simulink model "HighwayLaneFollowingTestBench"  (R2020a)
settings: Solver=ode23tb  StartTime=0.0  StopTime=scenario.StopTime  RelTol=1e-3
PostLoadFcn:
  | helperSLHighwayLaneFollowingSetup
values from neighbouring files (symbols this model uses):
  camera = obj.Camera    [HelperLaneMarkerDetector.m]    (also in HelperVisionVehicleDetector.m)
  m = hActors.Actors(n).ActorID.Data(sampleIndex)    [helperPlotLFDetectionResults.m]
  scenario = drivingScenario    [helperGetLaneFollowingScenario.m]
  vehSim3D = repmat(     struct(         'Length', 0,         'RearOverhang', 0,         'InitialPos',[0 0 0],         'InitialRot',[0 0 0]),     numVehicles,1)    [helperSLHighwayLaneFollowingSetup.m]
undefined symbols (not defined in the file or in its folder): actorProfiles, assessment, driving, lr, max_ac, max_dc, tau, tau2, Ts, v_set
libraries: drivingscenarioandsensors x9, sim3dautolib x6, simulink x4, helperCoordinateTransformLib x1, sim3dcameralib x1, sim3dprobsensorlib x1, sim3dlib x1, dspvision x1, autolibshared x1
CloseFcn:
  | helperSLHighwayLaneFollowingCleanUp
settings Model: SILPILModeSetting=veronly  SILPILSystemUnderTest=refmodels  Creator=The MathWorks, Inc.  LastModifiedBy=The MathWorks, Inc.
settings DataIOCC: SaveOutput=off  SaveTime=off  ReturnWorkspaceOutputs=off
settings DebuggingCC: ParameterPrecisionLossMsg=none  PregeneratedLibrarySubsystemCodeDiagnostic=none  ArithmeticOperatorsInVariantConditions=warning
settings HardwareCC: ProdLongLongMode=on
settings SFSimCC: SimUseLocalCustomCode=off
settings RTWCC: RTWUseLocalCustomCode=off
settings GRTTargetCC: RTWCAPISignals=on
settings ConfigComp: CovScope=ReferencedModels  CovIncludeTopModel=off

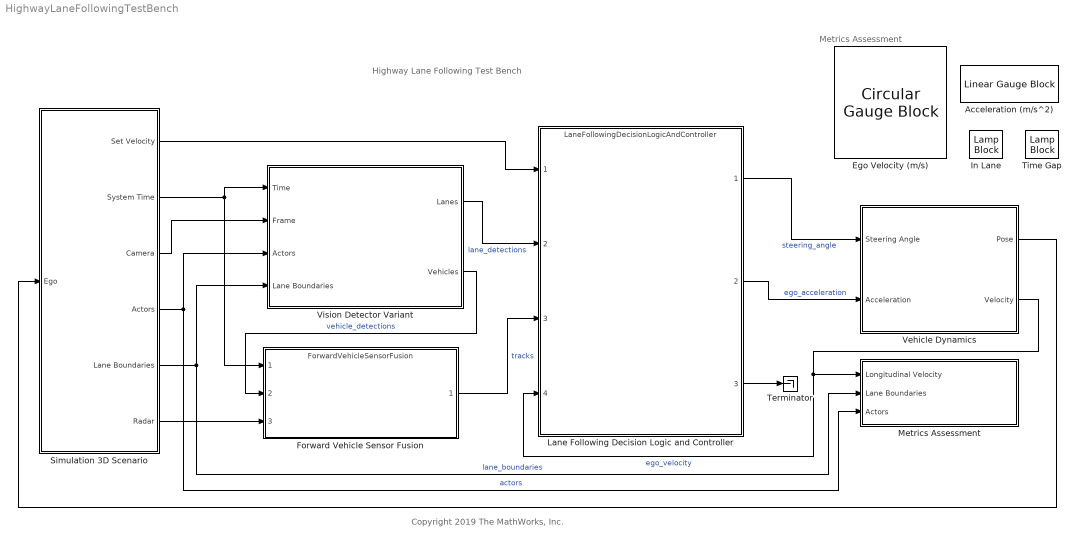
== system HighwayLaneFollowingTestBench ==
  note: Highway Lane Following Test Bench
  note: Metrics Assessment
  note: Copyright 2019 The MathWorks, Inc.
  Acceleration (m/s^2) : LinearGaugeBlock  LabelPosition=Hide  ScaleMin=-6  ScaleMax=6
  Ego Velocity (m/s) : CircularGaugeBlock  LabelPosition=Hide  ScaleMax=50
  Forward Vehicle Sensor Fusion : ModelReference  ModelNameDialog=ForwardVehicleSensorFusion.slx  SimulationMode=Normal  CodeInterface=Top model  ModelReferenceVersion=1.1423
  In Lane : LampBlock  LabelPosition=Hide
  Lane Following Decision Logic and Controller : ModelReference  ModelNameDialog=LaneFollowingDecisionLogicAndController.slx  SimulationMode=Normal  CodeInterface=Top model  ModelReferenceVersion=1.819
  Metrics Assessment : Subsystem
  Simulation 3D Scenario : Subsystem  VariantControl=1
  Terminator : Terminator
  Time Gap : LampBlock  LabelPosition=Hide
  Vehicle Dynamics : Subsystem  VariantControl=Variant2
  Vision Detector Variant : Subsystem  Variant=on
  wires:
  Vehicle Dynamics/2(Velocity) -> Metrics Assessment/1(Longitudinal Velocity), Lane Following Decision Logic and Controller/4  "ego_velocity"
  Simulation 3D Scenario/3(Camera) -> Vision Detector Variant/2(Frame)
  Simulation 3D Scenario/2(System Time) -> Vision Detector Variant/1(Time), Forward Vehicle Sensor Fusion/1
  Vehicle Dynamics/1(Pose) -> Simulation 3D Scenario/1(Ego)
  Simulation 3D Scenario/5(Lane Boundaries) -> Vision Detector Variant/4(Lane Boundaries), Metrics Assessment/2(Lane Boundaries)  "lane_boundaries"
  Simulation 3D Scenario/4(Actors) -> Metrics Assessment/3(Actors), Vision Detector Variant/3(Actors)  "actors"
  Lane Following Decision Logic and Controller/1 -> Vehicle Dynamics/1(Steering Angle)  "steering_angle"
  Simulation 3D Scenario/1(Set Velocity) -> Lane Following Decision Logic and Controller/1
  Lane Following Decision Logic and Controller/2 -> Vehicle Dynamics/2(Acceleration)  "ego_acceleration"
  Lane Following Decision Logic and Controller/3 -> Terminator/1
  Vision Detector Variant/1(Lanes) -> Lane Following Decision Logic and Controller/2  "lane_detections"
  Forward Vehicle Sensor Fusion/1 -> Lane Following Decision Logic and Controller/3  "tracks"
  Vision Detector Variant/2(Vehicles) -> Forward Vehicle Sensor Fusion/2  "vehicle_detections"
  Simulation 3D Scenario/6(Radar) -> Forward Vehicle Sensor Fusion/3

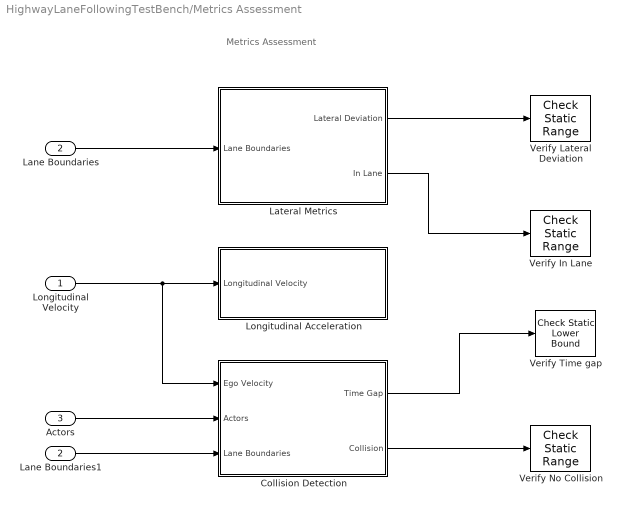
== system HighwayLaneFollowingTestBench/Metrics Assessment ==
  note: Metrics Assessment
  Longitudinal Velocity : Inport
  Lane Boundaries : Inport  Port=2
  Actors : Inport  Port=3
  Collision Detection : Subsystem
  Lane Boundaries1 : InportShadow  Port=2
  Lateral Metrics : Subsystem
  Longitudinal Acceleration : Subsystem
  Verify In Lane : simulink/Model Verification/Check  Static Range  Description=1 <= u <= 1  max=1  max_included=on  min=1  min_included=on  enabled=on  stopWhenAssertionFail=on  export=off  icon=graphic
      settings: SourceProductBaseCode=SL
  Verify Lateral Deviation : simulink/Model Verification/Check  Static Range  Description=-assessment.LateralDeviationMax <= u <= assessment.LateralDeviationMax  max=assessment.LateralDeviationMax  max_included=on  min=-assessment.LateralDeviationMax  min_included=on  enabled=on  stopWhenAssertionFail=on  export=off  icon=graphic
      settings: SourceProductBaseCode=SL
      settings: AttributesFormatString=|
      | ---------------------------------------
      | max = %<max>
      | min = %<min>
  Verify No Collision : simulink/Model Verification/Check  Static Range  Description=0 <= u <= 0  max=0  max_included=on  min=0  min_included=on  enabled=on  stopWhenAssertionFail=on  export=off  icon=graphic
      settings: SourceProductBaseCode=SL
  Verify Time gap : simulink/Model Verification/Check Static  Lower Bound  Description=assessment.TimeGap <= u  min=assessment.TimeGap  min_included=on  enabled=on  stopWhenAssertionFail=off  export=off  icon=graphic
      settings: AttributesFormatString=|
      | ---------------------------------------
      | min = %<min>
  wires:
  Actors/1 -> Collision Detection/2(Actors)
  Lateral Metrics/1(Lateral Deviation) -> Verify Lateral Deviation/1
  Collision Detection/1(Time Gap) -> Verify Time gap/1
  Collision Detection/2(Collision) -> Verify No Collision/1
  Longitudinal Velocity/1 -> Collision Detection/1(Ego Velocity), Longitudinal Acceleration/1(Longitudinal Velocity)
  Lane Boundaries/1 -> Lateral Metrics/1(Lane Boundaries)
  Lane Boundaries1/1 -> Collision Detection/3(Lane Boundaries)
  Lateral Metrics/2(In Lane) -> Verify In Lane/1

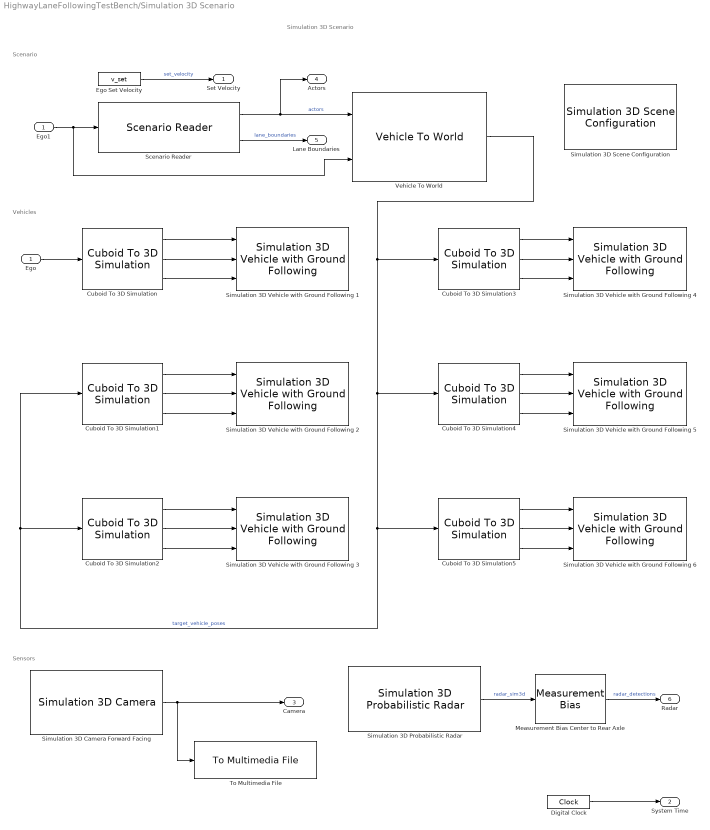
== system HighwayLaneFollowingTestBench/Simulation 3D Scenario ==
  note: Scenario
  note: Vehicles
  note: Simulation 3D Scenario
  note: Sensors
  Ego : Inport
  Cuboid To 3D Simulation : drivingscenarioandsensors/Cuboid To 3D Simulation  SpecifyActorID=off  ActorIDToConvert=1  SimulateUsing=Interpreted execution
      settings: SourceProductBaseCode=DR
  Cuboid To 3D Simulation1 : drivingscenarioandsensors/Cuboid To 3D Simulation  SpecifyActorID=on  ActorIDToConvert=2  SimulateUsing=Interpreted execution
      settings: SourceProductBaseCode=DR
  Cuboid To 3D Simulation2 : drivingscenarioandsensors/Cuboid To 3D Simulation  SpecifyActorID=on  ActorIDToConvert=3  SimulateUsing=Interpreted execution
      settings: SourceProductBaseCode=DR
  Cuboid To 3D Simulation3 : drivingscenarioandsensors/Cuboid To 3D Simulation  SpecifyActorID=on  ActorIDToConvert=4  SimulateUsing=Interpreted execution
      settings: SourceProductBaseCode=DR
  Cuboid To 3D Simulation4 : drivingscenarioandsensors/Cuboid To 3D Simulation  SpecifyActorID=on  ActorIDToConvert=5  SimulateUsing=Interpreted execution
      settings: SourceProductBaseCode=DR
  Cuboid To 3D Simulation5 : drivingscenarioandsensors/Cuboid To 3D Simulation  SpecifyActorID=on  ActorIDToConvert=6  SimulateUsing=Interpreted execution
      settings: SourceProductBaseCode=DR
  Digital Clock : DigitalClock  SampleTime=Ts
  Ego Set Velocity : Constant  Value=v_set  SampleTime=Ts
  Ego1 : InportShadow
  Measurement Bias Center to Rear Axle : helperCoordinateTransformLib/Measurement Bias  offsetPositionX=scenario.Actors(1).Length/2 - scenario.Actors(1).RearOverhang
      settings: AttributesFormatString=|
      | --------------------------------------
      | offsetPositionX =
      | %<offsetPositionX>
  Scenario Reader : drivingscenarioandsensors/Scenario Reader  ScenarioSource=From workspace  ScenarioFileName=dblLaneChangeDrivingScenario.mat  ScenarioVariableName=scenario  OutputCoordinateSystem=Vehicle coordinates  EgoVehicleSource=Input port  OrientVehiclesOnRoad=off  EgoVehicleActorID=1  OutputEgoVehiclePose=off  SampleTime=0.1  LaneBoundaryOutput=Ego vehicle lane boundaries  LaneBoundaryDistance=0:0.5:70  LaneBoundaryLocation=Center of lane markings  BusNameSource=Auto  BusName=BusActors  BusName2Source=Auto  BusName2=BusLaneBoundaries  BusName3Source=Auto  BusName3=BusEgoActor  ShowCoordinateLabels=on  SimulateUsing=Interpreted execution
  Simulation 3D Camera Forward Facing : sim3dcameralib/Simulation 3D Camera  Priority=1  sensorTag=Sim3dSensor1  sensorId=1  sensorName=Sim3dSensor1  vehTagList={'Scene Origin';'SimulinkVehicle1';'SimulinkVehicle4';'SimulinkVehicle5';'SimulinkVehicle6';'vehSim3D(2).InitialRot';'vehSim3D(3).InitialRot'}  vehTag=SimulinkVehicle1  mountLoc=Origin  offsetFlag=on  tmountOffset=camera.PositionSim3d  rmountOffset=camera.Rotation  FocalLength=camera.FocalLength  OpticalCenter=camera.PrincipalPoint  ImageSize=camera.ImageSize  RadialDistortion=[0, 0]  TangentialDistortion=[0, 0]  SensorSkew=0  DepthOutportEnabled=off  SemanticOutportEnabled=off  TransformOutportEnabled=off  SampleTime=-1  mountPoint=[0.57 0 1.2]  mountOrientation=[0 0 0]  aMode=3  ID=1
      settings: SourceProductBaseCode=DR,VE
      settings: AttributesFormatString=|
      | -------------------------------------
      | ImageSize = %<ImageSize>
      | OpticalCenter = %<OpticalCenter>
      | FocalLength = %<FocalLength>
      | RadialDistortion = %<RadialDistortion>
      | mountLoc = %<mountLoc>
      | tmountOffset = %<tmountOffset>
      | rmountOffset = %<rmountOffset>
      | Priority = %<Priority>
  Simulation 3D Probabilistic Radar : sim3dprobsensorlib/Simulation 3D Probabilistic Radar  Priority=1  sensorTag=Sim3dSensor2  sensorId=2  sensorName=Sim3dSensor2  vehTagList={'Scene Origin';'SimulinkVehicle1';'SimulinkVehicle4';'SimulinkVehicle5';'SimulinkVehicle6';'vehSim3D(2).InitialRot';'vehSim3D(3).InitialRot'}  vehTag=SimulinkVehicle1  mountLoc=Origin  offsetFlag=on  tmountOffset=radar.PositionSim3d  rmountOffset=radar.Rotation  AzimuthResolution=2  ElevationResolution=10  RangeResolution=2.5  RangeRateResolution=0.5  AzimuthBiasFraction=0.1  ElevationBiasFraction=0.1  RangeBiasFraction=0.05  RangeRateBiasFraction=0.05  FieldOfView=radar.FieldOfView  DetectionRange=radar.DetectionRanges  RangeRateLimits=[ -100, 100 ]  DetectionProbability=1  FalseAlarmRate=1e-6  ReferenceRange=100  ReferenceRCS=0  HasElevation=on  HasRangeRate=off  HasNoise=on  HasFalseAlarms=on  InitialSeedSource=Repeatable  InitialSeed=0  MaxNumDetections=50  DetectionCoordinates=Ego Cartesian  SpecifyOutputBusName=off  BusName=BusSimulation3DRadarTruthSensor  SampleTime=-1  mountPoint=[5.034 0 0.8]  mountOrientation=[0 0 0]  aMode=3  ID=2
      settings: SourceProductBaseCode=DR,VE
      settings: AttributesFormatString=|
      | -------------------------------------
      | FieldOfView = %<FieldOfView>
      | AzimuthResolution = %<AzimuthResolution>
      | DetectionCoordinates = %<DetectionCoordinates>
      | mountLoc = %<mountLoc>
      | tmountOffset = %<tmountOffset>
      | rmountOffset = %<rmountOffset>
      | Priority = %<Priority>
  Simulation 3D Scene Configuration : sim3dlib/Simulation 3D Scene Configuration  Priority=0  ProjectFormat=Default Scenes  SceneDesc=Curved road  ProjectName=VehicleSimulation.exe  ScenePath=/Game/Maps/HwStrght  vehTagList={'Scene Origin';'SimulinkVehicle1';'SimulinkVehicle4';'SimulinkVehicle5';'SimulinkVehicle6';'vehSim3D(2).InitialRot';'vehSim3D(3).InitialRot'}  vehTag=SimulinkVehicle1  OpVisEn=off  Ts=0.1  EnableWindow=on  sensorTag=MainCamera1  sensorId=1  sensorName=MainCamera1  mountLoc=Origin  offsetFlag=off  tmountOffset=[0, 0, 0]  rmountOffset=[0, 0, 0]  HorizontalResolution=1280  VerticalResolution=720  HorizontalFOV=60  mountPoint=[0 0 0]  mountOrientation=[0 0 0]  aMode=3  ID=1
      settings: SourceProductBaseCode=DR,VE
      settings: AttributesFormatString=|
      | -------------------------------------
      | SceneName = %<SceneDesc>
      | Priority = %<Priority>
  Simulation 3D Vehicle with Ground Following 1 : sim3dautolib/Simulation 3D Vehicle with Ground Following  Priority=-1  PassVehMesh=Sedan  VehColor=Blue  InitialPos=vehSim3D(1).InitialPos  InitialRot=vehSim3D(1).InitialRot  ActorName=SimulinkVehicle1  SampleTime=-1  ActorType=SimulinkVehicle  ID=1  aMode=3  ActorTag=SimulinkVehicle1  CoordinateScheme=ISO  TransformOutportEnabled=off
      settings: SourceProductBaseCode=DR,VE
      settings: AttributesFormatString=|
      | --------------------------------------
      | ActorName = %<ActorName>
      | PassVehMesh = %<PassVehMesh>
      | VehColor = %<VehColor>
      | InitialPos = %<InitialPos>
      | InitialRot = %<InitialRot>
      | Priority = %<Priority>
  Simulation 3D Vehicle with Ground Following 2 : sim3dautolib/Simulation 3D Vehicle with Ground Following  Priority=-1  PassVehMesh=Sedan  VehColor=Red  InitialPos=vehSim3D(2).InitialPos  InitialRot=vehSim3D(2).InitialRot  ActorName=vehSim3D(2).InitialRot  SampleTime=-1  ActorType=SimulinkVehicle  ID=C  aMode=3  ActorTag=vehSim3D(2).InitialRot  CoordinateScheme=ISO  TransformOutportEnabled=off
      settings: SourceProductBaseCode=DR,VE
      settings: AttributesFormatString=|
      | --------------------------------------
      | ActorName = %<ActorName>
      | PassVehMesh = %<PassVehMesh>
      | VehColor = %<VehColor>
      | InitialPos = %<InitialPos>
      | InitialRot = %<InitialRot>
      | Priority = %<Priority>
  Simulation 3D Vehicle with Ground Following 3 : sim3dautolib/Simulation 3D Vehicle with Ground Following  Priority=-1  PassVehMesh=Muscle car  VehColor=Black  InitialPos=vehSim3D(3).InitialPos  InitialRot=vehSim3D(3).InitialRot  ActorName=vehSim3D(3).InitialRot  SampleTime=-1  ActorType=SimulinkVehicle  ID=C  aMode=3  ActorTag=vehSim3D(3).InitialRot  CoordinateScheme=ISO  TransformOutportEnabled=off
      settings: SourceProductBaseCode=DR,VE
      settings: AttributesFormatString=|
      | --------------------------------------
      | ActorName = %<ActorName>
      | PassVehMesh = %<PassVehMesh>
      | VehColor = %<VehColor>
      | InitialPos = %<InitialPos>
      | InitialRot = %<InitialRot>
      | Priority = %<Priority>
  Simulation 3D Vehicle with Ground Following 4 : sim3dautolib/Simulation 3D Vehicle with Ground Following  Priority=-1  PassVehMesh=Hatchback  VehColor=Orange  InitialPos=vehSim3D(4).InitialPos  InitialRot=vehSim3D(4).InitialRot  ActorName=SimulinkVehicle4  SampleTime=-1  ActorType=SimulinkVehicle  ID=4  aMode=3  ActorTag=SimulinkVehicle4  CoordinateScheme=ISO  TransformOutportEnabled=off
      settings: SourceProductBaseCode=DR,VE
      settings: AttributesFormatString=|
      | --------------------------------------
      | ActorName = %<ActorName>
      | PassVehMesh = %<PassVehMesh>
      | VehColor = %<VehColor>
      | InitialPos = %<InitialPos>
      | InitialRot = %<InitialRot>
      | Priority = %<Priority>
  Simulation 3D Vehicle with Ground Following 5 : sim3dautolib/Simulation 3D Vehicle with Ground Following  Priority=-1  PassVehMesh=Small pickup truck  VehColor=Green  InitialPos=vehSim3D(5).InitialPos  InitialRot=vehSim3D(5).InitialRot  ActorName=SimulinkVehicle5  SampleTime=-1  ActorType=SimulinkVehicle  ID=5  aMode=3  ActorTag=SimulinkVehicle5  CoordinateScheme=ISO  TransformOutportEnabled=off
      settings: SourceProductBaseCode=DR,VE
      settings: AttributesFormatString=|
      | --------------------------------------
      | ActorName = %<ActorName>
      | PassVehMesh = %<PassVehMesh>
      | VehColor = %<VehColor>
      | InitialPos = %<InitialPos>
      | InitialRot = %<InitialRot>
      | Priority = %<Priority>
  Simulation 3D Vehicle with Ground Following 6 : sim3dautolib/Simulation 3D Vehicle with Ground Following  Priority=-1  PassVehMesh=Sport utility vehicle  VehColor=Blue  InitialPos=vehSim3D(6).InitialPos  InitialRot=vehSim3D(6).InitialRot  ActorName=SimulinkVehicle6  SampleTime=-1  ActorType=SimulinkVehicle  ID=6  aMode=3  ActorTag=SimulinkVehicle6  CoordinateScheme=ISO  TransformOutportEnabled=off
      settings: SourceProductBaseCode=DR,VE
      settings: AttributesFormatString=|
      | --------------------------------------
      | ActorName = %<ActorName>
      | PassVehMesh = %<PassVehMesh>
      | VehColor = %<VehColor>
      | InitialPos = %<InitialPos>
      | InitialRot = %<InitialRot>
      | Priority = %<Priority>
  To Multimedia File : dspvision/To Multimedia File  outputFilename=forwardFacingCamera.mp4  streamSelection=Video only  videoCompressor=None (uncompressed)  audioCompressor=None (uncompressed)  imagePorts=One multidimensional signal  fileType=MPEG4  audioDatatype=Determine from input data type  fourcc=RGB  videoQuality=75  mj2000CompFactor=10
  Vehicle To World : drivingscenarioandsensors/Vehicle To World  BusNameSource=Auto  BusName=BusVehicleToWorldActors  SimulateUsing=Interpreted execution
      settings: SourceProductBaseCode=DR
  Set Velocity : Outport  Unit=m/s  VectorParamsAs1DForOutWhenUnconnected=off
  System Time : Outport  Port=2  VectorParamsAs1DForOutWhenUnconnected=off
  Camera : Outport  Port=3  VectorParamsAs1DForOutWhenUnconnected=off
  Actors : Outport  Port=4
  Lane Boundaries : Outport  Port=5
  Radar : Outport  Port=6  VectorParamsAs1DForOutWhenUnconnected=off
  wires:
  Digital Clock/1 -> System Time/1
  Cuboid To 3D Simulation/2 -> Simulation 3D Vehicle with Ground Following 1/2
  Cuboid To 3D Simulation/1 -> Simulation 3D Vehicle with Ground Following 1/1
  Cuboid To 3D Simulation/3 -> Simulation 3D Vehicle with Ground Following 1/3
  Ego/1 -> Cuboid To 3D Simulation/1
  Cuboid To 3D Simulation1/2 -> Simulation 3D Vehicle with Ground Following 2/2
  Cuboid To 3D Simulation1/1 -> Simulation 3D Vehicle with Ground Following 2/1
  Cuboid To 3D Simulation1/3 -> Simulation 3D Vehicle with Ground Following 2/3
  Simulation 3D Probabilistic Radar/1 -> Measurement Bias Center to Rear Axle/1  "radar_sim3d"
  Simulation 3D Camera Forward Facing/1 -> Camera/1, To Multimedia File/1
  Measurement Bias Center to Rear Axle/1 -> Radar/1  "radar_detections"
  Scenario Reader/1 -> Vehicle To World/1, Actors/1  "actors"
  Vehicle To World/1 -> Cuboid To 3D Simulation3/1, Cuboid To 3D Simulation4/1, Cuboid To 3D Simulation5/1, Cuboid To 3D Simulation2/1, Cuboid To 3D Simulation1/1  "target_vehicle_poses"
  Cuboid To 3D Simulation3/2 -> Simulation 3D Vehicle with Ground Following 4/2
  Cuboid To 3D Simulation3/3 -> Simulation 3D Vehicle with Ground Following 4/3
  Cuboid To 3D Simulation2/2 -> Simulation 3D Vehicle with Ground Following 3/2
  Cuboid To 3D Simulation3/1 -> Simulation 3D Vehicle with Ground Following 4/1
  Cuboid To 3D Simulation2/3 -> Simulation 3D Vehicle with Ground Following 3/3
  Cuboid To 3D Simulation2/1 -> Simulation 3D Vehicle with Ground Following 3/1
  Cuboid To 3D Simulation4/3 -> Simulation 3D Vehicle with Ground Following 5/3
  Cuboid To 3D Simulation5/2 -> Simulation 3D Vehicle with Ground Following 6/2
  Cuboid To 3D Simulation5/3 -> Simulation 3D Vehicle with Ground Following 6/3
  Cuboid To 3D Simulation5/1 -> Simulation 3D Vehicle with Ground Following 6/1
  Cuboid To 3D Simulation4/2 -> Simulation 3D Vehicle with Ground Following 5/2
  Cuboid To 3D Simulation4/1 -> Simulation 3D Vehicle with Ground Following 5/1
  Scenario Reader/2 -> Lane Boundaries/1  "lane_boundaries"
  Ego1/1 -> Vehicle To World/2, Scenario Reader/1
  Ego Set Velocity/1 -> Set Velocity/1  "set_velocity"

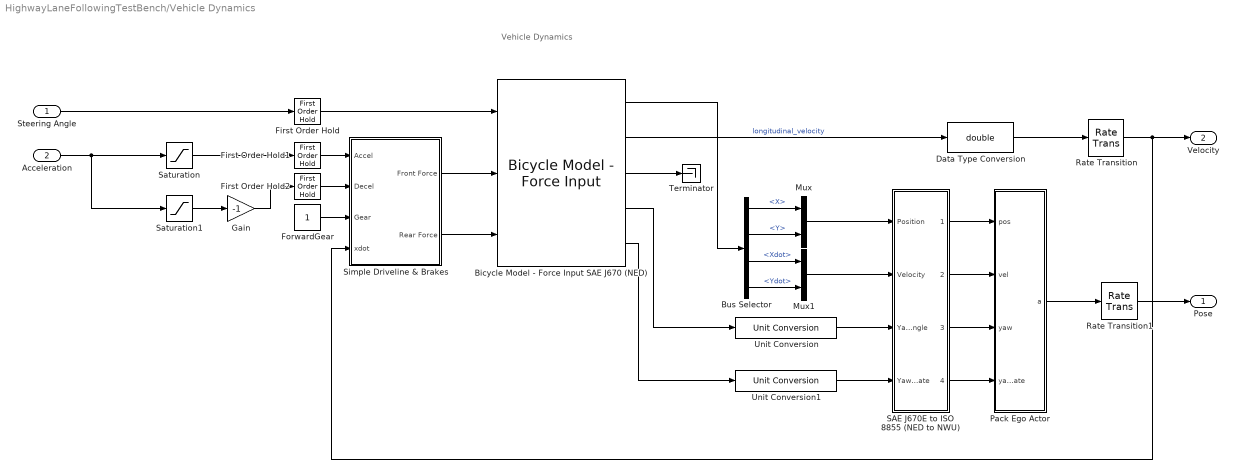
== system HighwayLaneFollowingTestBench/Vehicle Dynamics ==
  note: Vehicle Dynamics
  Steering Angle : Inport  Unit=rad
  Acceleration : Inport  Port=2  Unit=m/s^2
  Bicycle Model - Force Input SAE J670 (NED) : autolibshared/Bicycle Model - Force Input  trackMode=Single (bicycle)  inputMode=External longitudinal forces  frontSteerMode=on  rearSteerMode=off  windMode=off  muMode=off  extFMode=off  extMMode=off  aMode=3  NF=2  NR=2  m=m  a=lf  b=lr  h=0.35  X_o=egoVehDyn.X0  xdot_o=egoVehDyn.VLong0  CalphaMode=off  sigmaMode=on  w=[1.4,1.4]  Cy_f=Cf  Cy_r=Cr  sigma_f=.1  sigma_r=.1  alpha_f_brk=[-.1 .1]  Cy_f_data=[-9e3 9e3]  alpha_r_brk=[-.1 .1]  Cy_r_data=[-9e3 9e3]  Y_o=egoVehDyn.Y0  ydot_o=0  Izz=Iz  psi_o=egoVehDyn.Yaw0  r_o=0  Af=0  Cd=.3  Cl=.1  Cpm=.1  beta_w=[0:0.01:0.3]  Cs=[0:0.03:0.9]  Cym=[0:0.01:0.3]  Pabs=101325  Tair=273  g=9.81  mu=1  xdot_tol=.01  Fznom=5000  Fxtire_sat=1e6  Fytire_sat=1e6  longOff=0  latOff=0  vertOff=0
      settings: SourceProductBaseCode=PW,MT,VE,VP
      settings: AttributesFormatString=|
      | ---------------------------------
      | X_o = %<X_o>
      | Y_o = %<Y_o>
      | psi_o = %<psi_o>
      | xdot_o = %<xdot_o>
      | ydot_o = %<ydot_o>
  Bus Selector : BusSelector  OutputSignals=InertFrm.RearAxl.Disp.X,InertFrm.RearAxl.Disp.Y,InertFrm.RearAxl.Vel.Xdot,InertFrm.RearAxl.Vel.Ydot
  Data Type Conversion : DataTypeConversion  OutDataTypeStr=double
  First Order Hold : FirstOrderHold  ErrorTolerance=inf
  First Order Hold1 : FirstOrderHold  ErrorTolerance=inf
  First Order Hold2 : FirstOrderHold  ErrorTolerance=inf
  ForwardGear : Constant  SampleTime=Ts
  Gain : Gain  Gain=-1
  Mux : Mux  Inputs=2
  Mux1 : Mux  Inputs=2
  Pack Ego Actor : MATLAB Function  TreatAsAtomicUnit=on
  Rate Transition : RateTransition
  Rate Transition1 : RateTransition
  SAE J670E to ISO 8855 (NED to NWU) : Subsystem
  Saturation : Saturate  UpperLimit=max_ac  LowerLimit=0
  Saturation1 : Saturate  UpperLimit=0  LowerLimit=max_dc
  Simple Driveline & Brakes : Subsystem
  Terminator : Terminator
  Unit Conversion : UnitConversion  OutputType=Inherit: Inherit via back propagation
  Unit Conversion1 : UnitConversion  OutputType=Inherit: Inherit via back propagation
  Pose : Outport  VectorParamsAs1DForOutWhenUnconnected=off
  Velocity : Outport  Port=2  Unit=m/s  VectorParamsAs1DForOutWhenUnconnected=off
  wires:
  Bicycle Model - Force Input SAE J670 (NED)/2 -> Data Type Conversion/1  "longitudinal_velocity"
  Steering Angle/1 -> First Order Hold/1
  Rate Transition/1 -> Simple Driveline & Brakes/4(xdot), Velocity/1
  Bus Selector/3 -> Mux1/1  "<Xdot>"
  Bicycle Model - Force Input SAE J670 (NED)/1 -> Bus Selector/1
  SAE J670E to ISO 8855 (NED to NWU)/4(4) -> Pack Ego Actor/4(yawRate)
  Bicycle Model - Force Input SAE J670 (NED)/5 -> Unit Conversion1/1
  SAE J670E to ISO 8855 (NED to NWU)/3(3) -> Pack Ego Actor/3(yaw)
  Bus Selector/1 -> Mux/1  "<X>"
  Mux/1 -> SAE J670E to ISO 8855 (NED to NWU)/1(Position)
  Pack Ego Actor/1(a) -> Rate Transition1/1
  Bus Selector/2 -> Mux/2  "<Y>"
  Bicycle Model - Force Input SAE J670 (NED)/4 -> Unit Conversion/1
  Mux1/1 -> SAE J670E to ISO 8855 (NED to NWU)/2(Velocity)
  SAE J670E to ISO 8855 (NED to NWU)/2(2) -> Pack Ego Actor/2(vel)
  Unit Conversion1/1 -> SAE J670E to ISO 8855 (NED to NWU)/4(Yaw Rate)
  Bus Selector/4 -> Mux1/2  "<Ydot>"
  Unit Conversion/1 -> SAE J670E to ISO 8855 (NED to NWU)/3(Yaw Angle)
  SAE J670E to ISO 8855 (NED to NWU)/1(1) -> Pack Ego Actor/1(pos)
  Rate Transition1/1 -> Pose/1
  Bicycle Model - Force Input SAE J670 (NED)/3 -> Terminator/1
  ForwardGear/1 -> Simple Driveline & Brakes/3(Gear)
  Simple Driveline & Brakes/1(Front Force) -> Bicycle Model - Force Input SAE J670 (NED)/2
  Simple Driveline & Brakes/2(Rear Force) -> Bicycle Model - Force Input SAE J670 (NED)/3
  Data Type Conversion/1 -> Rate Transition/1
  First Order Hold/1 -> Bicycle Model - Force Input SAE J670 (NED)/1
  First Order Hold1/1 -> Simple Driveline & Brakes/1(Accel)
  First Order Hold2/1 -> Simple Driveline & Brakes/2(Decel)
  Saturation/1 -> First Order Hold1/1
  Acceleration/1 -> Saturation1/1, Saturation/1
  Saturation1/1 -> Gain/1
  Gain/1 -> First Order Hold2/1

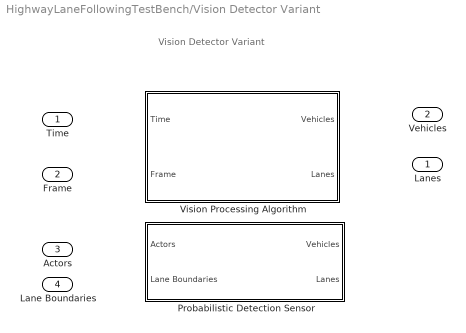
== system HighwayLaneFollowingTestBench/Vision Detector Variant ==
  note: Vision Detector Variant
  Time : Inport
  Frame : Inport  Port=2
  Actors : Inport  Port=3
  Lane Boundaries : Inport  Port=4
  Probabilistic Detection Sensor : Subsystem  VariantControl="visionVariant == \"ProbabilisticDetectionSensor\""
  Vision Processing Algorithm : Subsystem  VariantControl="visionVariant == \"VisionProcessingAlgorithm\""
  Lanes : Outport
  Vehicles : Outport  Port=2

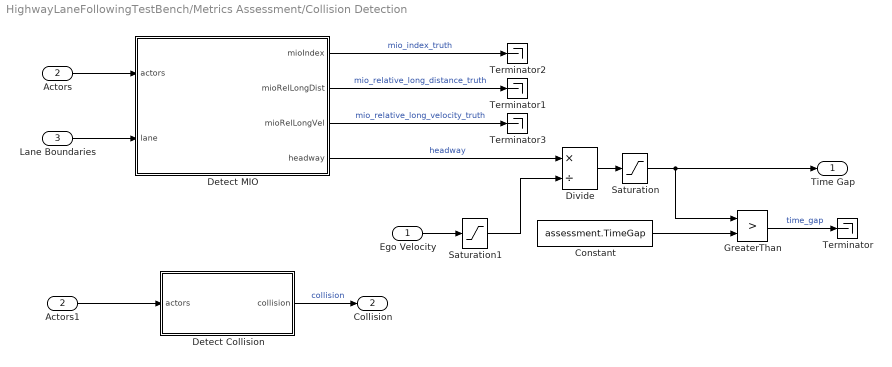
== system HighwayLaneFollowingTestBench/Metrics Assessment/Collision Detection ==
  Ego Velocity : Inport
  Actors : Inport  Port=2
  Lane Boundaries : Inport  Port=3
  Actors1 : InportShadow  Port=2
  Constant : Constant  Value=assessment.TimeGap
  Detect Collision : MATLAB Function  TreatAsAtomicUnit=on  mask(Detect Collision){vehicleProfiles=actorProfiles(scenario)}
      mask prompts: vehicleProfiles "Vehicle profiles"
      mask help:
      | Detect collision between ego and target vehicles.
      | Vehicle profiles is expected to be the struture returned by the actorProfiles method of a drivingScenerio object.
      settings: AttributesFormatString=|
      | ------------------------------------------
      | vehicleProfiles = %<vehicleProfiles>
  Detect MIO : MATLAB Function  TreatAsAtomicUnit=on  mask(Detect Most Important Obejct (MIO)){vehicleProfiles=actorProfiles(scenario)}
      mask prompts: vehicleProfiles "Vehicle profiles"
      mask help:
      | Detect most important object (MIO) in ego vehicle lane.
      | Headway to MIO takes into account the vehicel dimensions.
      | Vehicle profiles is expected to be the struture returned by the actorProfiles method of a drivingScenerio object.
      settings: AttributesFormatString=|
      | ------------------------------------------
      | vehicleProfiles = %<vehicleProfiles>
  Divide : Product  Inputs=*/
  GreaterThan : RelationalOperator  Operator=>  OutDataTypeStr=boolean  RndMeth=Simplest
  Saturation : Saturate  UpperLimit=4  LowerLimit=0
  Saturation1 : Saturate  UpperLimit=100  LowerLimit=0.01
  Terminator{,1..3} (4 alike) : Terminator
  Time Gap : Outport
  Collision : Outport  Port=2
  wires:
  Actors/1 -> Detect MIO/1(actors)
  Lane Boundaries/1 -> Detect MIO/2(lane)
  Detect MIO/4(headway) -> Divide/1  "headway"
  Ego Velocity/1 -> Saturation1/1
  Divide/1 -> Saturation/1
  Saturation/1 -> Time Gap/1, GreaterThan/1
  Saturation1/1 -> Divide/2
  Constant/1 -> GreaterThan/2
  GreaterThan/1 -> Terminator/1  "time_gap"
  Detect MIO/2(mioRelLongDist) -> Terminator1/1  "mio_relative_long_distance_truth"
  Detect MIO/1(mioIndex) -> Terminator2/1  "mio_index_truth"
  Detect Collision/1(collision) -> Collision/1  "collision"
  Detect MIO/3(mioRelLongVel) -> Terminator3/1  "mio_relative_long_velocity_truth"
  Actors1/1 -> Detect Collision/1(actors)

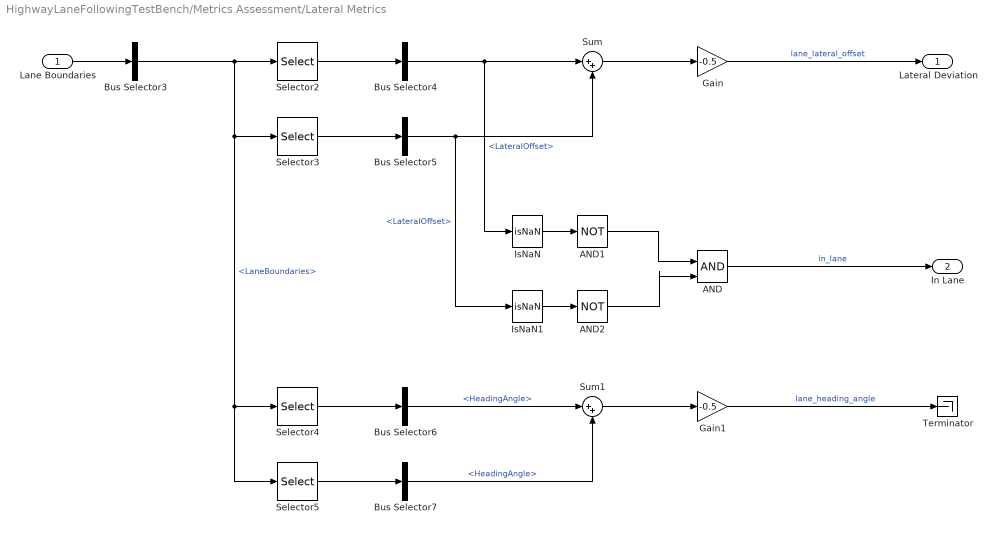
== system HighwayLaneFollowingTestBench/Metrics Assessment/Lateral Metrics ==
  Lane Boundaries : Inport
  AND : Logic  IconShape=distinctive  AllPortsSameDT=off  OutDataTypeStr=boolean
  AND1 : Logic  Operator=NOT  IconShape=distinctive  AllPortsSameDT=off  OutDataTypeStr=boolean
  AND2 : Logic  Operator=NOT  IconShape=distinctive  AllPortsSameDT=off  OutDataTypeStr=boolean
  Bus Selector3 : BusSelector  OutputSignals=LaneBoundaries
  Bus Selector4 : BusSelector  OutputSignals=LateralOffset
  Bus Selector5 : BusSelector  OutputSignals=LateralOffset
  Bus Selector6 : BusSelector  OutputSignals=HeadingAngle
  Bus Selector7 : BusSelector  OutputSignals=HeadingAngle
  Gain : Gain  Gain=-0.5
  Gain1 : Gain  Gain=-0.5
  IsNaN : RelationalOperator  Operator=isNaN  OutDataTypeStr=boolean  RndMeth=Simplest
  IsNaN1 : RelationalOperator  Operator=isNaN  OutDataTypeStr=boolean  RndMeth=Simplest
  Selector2 : Selector  InputPortWidth=2  IndexOptions=Index vector (dialog)  Indices=1  OutputSizes=1
  Selector3 : Selector  InputPortWidth=2  IndexOptions=Index vector (dialog)  Indices=2  OutputSizes=1
  Selector4 : Selector  InputPortWidth=2  IndexOptions=Index vector (dialog)  Indices=1  OutputSizes=1
  Selector5 : Selector  InputPortWidth=2  IndexOptions=Index vector (dialog)  Indices=2  OutputSizes=1
  Sum : Sum  Inputs=|++
  Sum1 : Sum  Inputs=|++
  Terminator : Terminator
  Lateral Deviation : Outport  VectorParamsAs1DForOutWhenUnconnected=off
  In Lane : Outport  Port=2
  wires:
  AND/1 -> In Lane/1  "in_lane"
  IsNaN1/1 -> AND2/1
  IsNaN/1 -> AND1/1
  Sum/1 -> Gain/1
  Bus Selector5/1 -> IsNaN1/1, Sum/2  "<LateralOffset>"
  Selector2/1 -> Bus Selector4/1
  Bus Selector4/1 -> IsNaN/1, Sum/1  "<LateralOffset>"
  Selector3/1 -> Bus Selector5/1
  Lane Boundaries/1 -> Bus Selector3/1
  Gain/1 -> Lateral Deviation/1  "lane_lateral_offset"
  AND1/1 -> AND/1
  AND2/1 -> AND/2
  Selector5/1 -> Bus Selector7/1
  Bus Selector6/1 -> Sum1/1  "<HeadingAngle>"
  Selector4/1 -> Bus Selector6/1
  Bus Selector3/1 -> Selector2/1, Selector3/1, Selector4/1, Selector5/1  "<LaneBoundaries>"
  Sum1/1 -> Gain1/1
  Bus Selector7/1 -> Sum1/2  "<HeadingAngle>"
  Gain1/1 -> Terminator/1  "lane_heading_angle"

== system HighwayLaneFollowingTestBench/Metrics Assessment/Longitudinal Acceleration ==
  Longitudinal Velocity : Inport
  Derivative : Derivative
  Terminator : Terminator
  wires:
  Derivative/1 -> Terminator/1  "longitudinal_acceleration"
  Longitudinal Velocity/1 -> Derivative/1

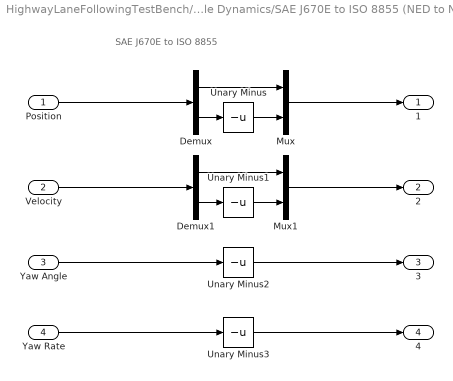
== system HighwayLaneFollowingTestBench/Vehicle Dynamics/SAE J670E to ISO 8855 (NED to NWU) ==
  note: SAE J670E to ISO 8855
  Position : Inport  Unit=m
  Velocity : Inport  Port=2  Unit=m/s
  Yaw Angle : Inport  Port=3  Unit=deg
  Yaw Rate : Inport  Port=4  Unit=deg/s
  Demux : Demux  Outputs=2
  Demux1 : Demux  Outputs=2
  Mux : Mux  Inputs=2
  Mux1 : Mux  Inputs=2
  Unary Minus{,1..3} (4 alike) : UnaryMinus
  1 : Outport  VectorParamsAs1DForOutWhenUnconnected=off
  2 : Outport  Port=2  VectorParamsAs1DForOutWhenUnconnected=off
  3 : Outport  Port=3  VectorParamsAs1DForOutWhenUnconnected=off
  4 : Outport  Port=4  VectorParamsAs1DForOutWhenUnconnected=off
  wires:
  Yaw Rate/1 -> Unary Minus3/1
  Yaw Angle/1 -> Unary Minus2/1
  Demux/1 -> Mux/1
  Demux/2 -> Unary Minus/1
  Unary Minus/1 -> Mux/2
  Unary Minus1/1 -> Mux1/2
  Demux1/2 -> Unary Minus1/1
  Demux1/1 -> Mux1/1
  Mux1/1 -> 2/1
  Mux/1 -> 1/1
  Position/1 -> Demux/1
  Velocity/1 -> Demux1/1
  Unary Minus2/1 -> 3/1
  Unary Minus3/1 -> 4/1

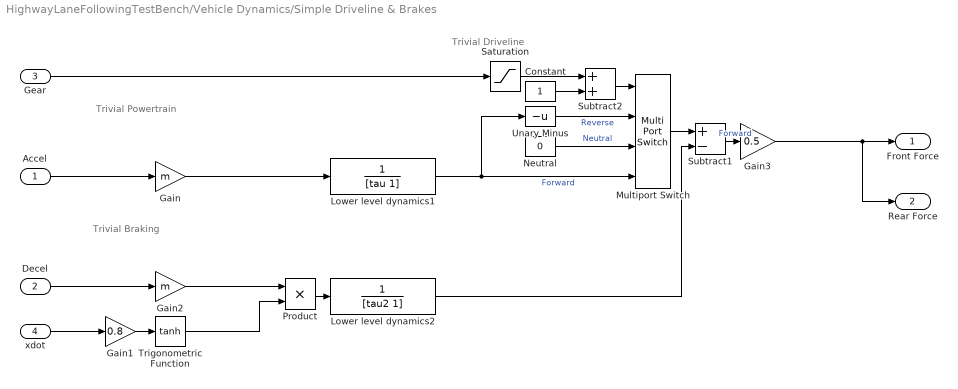
== system HighwayLaneFollowingTestBench/Vehicle Dynamics/Simple Driveline & Brakes ==
  note: Trivial Driveline
  note: Trivial Powertrain
  note: Trivial Braking
  Accel : Inport
  Decel : Inport  Port=2
  Gear : Inport  Port=3
  xdot : Inport  Port=4
  Constant : Constant
  Gain : Gain  Gain=m
  Gain1 : Gain  Gain=0.8
  Gain2 : Gain  Gain=m
  Gain3 : Gain  Gain=0.5
  Lower level dynamics1 : TransferFcn  Denominator=[tau 1]
  Lower level dynamics2 : TransferFcn  Denominator=[tau2 1]
  Multiport Switch : MultiPortSwitch  DataPortOrder=Zero-based contiguous  zeroidx=on
  Neutral : Constant  Value=0
  Product : Product
  Saturation : Saturate  UpperLimit=1  LowerLimit=-1  ZeroCross=off
  Subtract1 : Sum  Inputs=+-
  Subtract2 : Sum
  Trigonometric Function : Trigonometry  Operator=tanh
  Unary Minus : UnaryMinus
  Front Force : Outport  VectorParamsAs1DForOutWhenUnconnected=off
  Rear Force : Outport  Port=2  VectorParamsAs1DForOutWhenUnconnected=off
  wires:
  Multiport Switch/1 -> Subtract1/1
  Accel/1 -> Gain/1
  xdot/1 -> Gain1/1
  Decel/1 -> Gain2/1
  Trigonometric Function/1 -> Product/2
  Gain1/1 -> Trigonometric Function/1
  Gain/1 -> Lower level dynamics1/1
  Gain2/1 -> Product/1
  Lower level dynamics2/1 -> Subtract1/2
  Product/1 -> Lower level dynamics2/1
  Gear/1 -> Saturation/1
  Constant/1 -> Subtract2/2
  Subtract2/1 -> Multiport Switch/1
  Neutral/1 -> Multiport Switch/3  "Neutral"
  Lower level dynamics1/1 -> Unary Minus/1, Multiport Switch/4  "Forward"
  Saturation/1 -> Subtract2/1
  Subtract1/1 -> Gain3/1  "Forward"
  Unary Minus/1 -> Multiport Switch/2  "Reverse"
  Gain3/1 -> Front Force/1, Rear Force/1

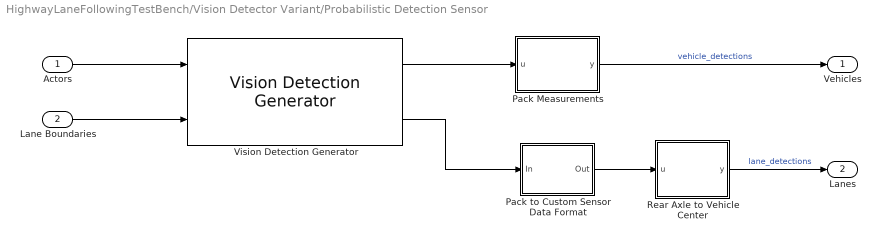
== system HighwayLaneFollowingTestBench/Vision Detector Variant/Probabilistic Detection Sensor ==
  Actors : Inport
  Lane Boundaries : Inport  Port=2
  "Pack Measurements " : MATLAB Function  TreatAsAtomicUnit=on  mask(Pack vision detections){structInit=Simulink.Bus.createMATLABStruct('BusVision'), measurementNoise=camera.MeasurementNoise}
      mask prompts: structInit "Output struct"; measurementNoise "Measurement noise"
      mask help: Packs vision detections to match bus used by vision processing algorithm. This includes replacing the measurement noise and disabling the velocity measurement.
  Pack to Custom Sensor Data Format : Subsystem
  Rear Axle to Vehicle Center : MATLAB Function  TreatAsAtomicUnit=on  mask(Shift lateral offset){offsetX=camera.Position(1) - camera.PositionSim3d(1)}
      mask prompts: offsetX "Offset"
      mask help:
      | Lateral offset output from Vision Detection Generator is with respect to vehicle rear axle. The lateral controller expects the lateral offset to be with respect to vehicle center. The offset to shift the lateral offset is calculated as:
      |
      |   camera position (with respect to rear axle)
      | - camera position (with repect to vehicle center)
  Vision Detection Generator : drivingscenarioandsensors/Vision Detection Generator  SensorIndex=1  DetectorOutput=Lanes and objects  UpdateInterval=Ts  LaneUpdateInterval=Ts  SensorLocation=camera.Position([1,2])  Height=camera.Position(3)  Yaw=camera.Rotation(3)  Pitch=camera.Rotation(2)  Roll=camera.Rotation(1)  BusNameSource=Auto  BusName=BusVision  BusName2Source=Auto  BusName2=BusLanes  MaxNumDetectionsSource=Property  MaxNumDetections=20  MaxNumLanesSource=Property  MaxNumLanes=2  DetectionCoordinates=Ego Cartesian  SimulateUsing=Interpreted execution  MaxRange=camera.DetectionRanges(2)  BoundingBoxAccuracy=5  ProcessNoiseIntensity=5  MaxSpeed=50  MaxAllowedOcclusion=0.5  MinObjectImageSize=camera.MinObjectImageSize  DetectionProbability=0.9  FalsePositivesPerImage=0  MinLaneImageSize=[ 20, 3 ]  LaneBoundaryAccuracy=3  HasNoise=on  InitialSeedSource=Repeatable  InitialSeed=0  UsedSeed=driving.internal.SimulinkUtilities.seedManager(gcb)  ActorProfilesSource=MATLAB expression  ActorProfilesParameters=driving.internal.ActorProfilesParameters  ActorProfilesExpression=actorProfiles(scenario)  Intrinsics=driving.internal.cameraIntrinsics('FocalLength',camera.FocalLength,'ImageSize',camera.ImageSize,'PrincipalPoint',camera.PrincipalPoint)
      settings: AttributesFormatString=|
      | ----------------------------------
      | SensorLocation = %<SensorLocation>
      | Height = %<Height>
      | Roll = %<Roll>
      | Pitch = %<Pitch>
      | Yaw = %<Yaw>
      | MaxRange = %<MaxRange>
      | MinObjectImageSize = %<MinObjectImageSize>
  Vehicles : Outport
  Lanes : Outport  Port=2
  wires:
  "Pack Measurements "/1(y) -> Vehicles/1  "vehicle_detections"
  Rear Axle to Vehicle Center/1(y) -> Lanes/1  "lane_detections"
  Vision Detection Generator/2 -> Pack to Custom Sensor Data Format/1(In)
  Vision Detection Generator/1 -> "Pack Measurements "/1(u)
  Lane Boundaries/1 -> Vision Detection Generator/2
  Actors/1 -> Vision Detection Generator/1
  Pack to Custom Sensor Data Format/1(Out) -> Rear Axle to Vehicle Center/1(u)

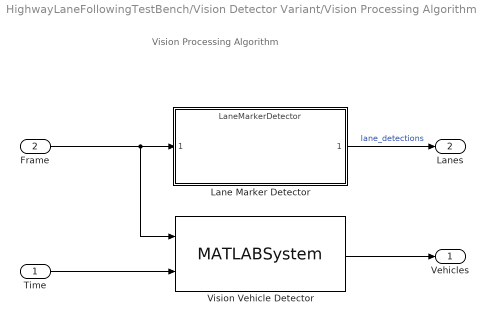
== system HighwayLaneFollowingTestBench/Vision Detector Variant/Vision Processing Algorithm ==
  note: Vision Processing Algorithm
  Time : Inport
  Frame : Inport  Port=2
  Lane Marker Detector : ModelReference  ModelNameDialog=LaneMarkerDetector.slx  SimulationMode=Normal  CodeInterface=Top model  ModelReferenceVersion=1.1577
  Vision Vehicle Detector : MATLABSystem  System=HelperVisionVehicleDetector  EnableVehicleDetector=on  EnableDisplay=on  Camera=camera
      mask Type: HelperVisionVehicleDetector
      mask Display:
      | disp('HelperVisionVehicleDetector');
      | port_label('input',1,'frame');
      | port_label('input',2,'t');
      | port_label('output',1,'vehicles');
  Vehicles : Outport
  Lanes : Outport  Port=2
  wires:
  Vision Vehicle Detector/1 -> Vehicles/1
  Time/1 -> Vision Vehicle Detector/2
  Frame/1 -> Vision Vehicle Detector/1, Lane Marker Detector/1
  Lane Marker Detector/1 -> Lanes/1  "lane_detections"

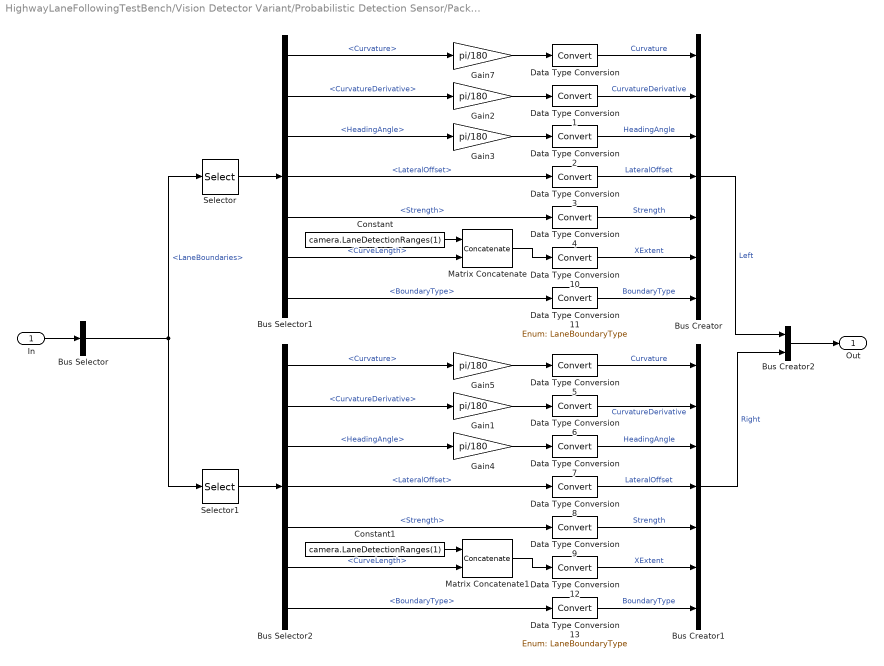
== system HighwayLaneFollowingTestBench/Vision Detector Variant/Probabilistic Detection Sensor/Pack to Custom Sensor Data Format ==
  In : Inport
  Bus Creator : BusCreator  Inputs=7  OutDataTypeStr=Bus: LaneSensorBoundaries
  Bus Creator1 : BusCreator  Inputs=7  OutDataTypeStr=Bus: LaneSensorBoundaries
  Bus Creator2 : BusCreator  Inputs=2  OutDataTypeStr=Bus: LaneSensor
  Bus Selector : BusSelector  OutputSignals=LaneBoundaries
  Bus Selector1 : BusSelector  OutputSignals=Curvature,CurvatureDerivative,HeadingAngle,LateralOffset,Strength,CurveLength,BoundaryType
  Bus Selector2 : BusSelector  OutputSignals=Curvature,CurvatureDerivative,HeadingAngle,LateralOffset,Strength,CurveLength,BoundaryType
  Constant : Constant  Value=camera.LaneDetectionRanges(1)
  Constant1 : Constant  Value=camera.LaneDetectionRanges(1)
  Data Type Conversion{,1..10,12} (12 alike) : DataTypeConversion
  Data Type Conversion11 : DataTypeConversion  OutDataTypeStr=Enum: LaneBoundaryType
  Data Type Conversion13 : DataTypeConversion  OutDataTypeStr=Enum: LaneBoundaryType
  Gain{1..5,7} (6 alike) : Gain  Gain=pi/180
  Matrix Concatenate : Concatenate  Mode=Multidimensional array  ConcatenateDimension=2
  Matrix Concatenate1 : Concatenate  Mode=Multidimensional array  ConcatenateDimension=2
  Selector : Selector  InputPortWidth=2  IndexOptions=Index vector (dialog)  Indices=1  OutputSizes=1
  Selector1 : Selector  InputPortWidth=2  IndexOptions=Index vector (dialog)  Indices=2  OutputSizes=1
  Out : Outport  VectorParamsAs1DForOutWhenUnconnected=off
  wires:
  In/1 -> Bus Selector/1
  Bus Selector/1 -> Selector/1, Selector1/1  "<LaneBoundaries>"
  Selector/1 -> Bus Selector1/1
  Bus Selector1/2 -> Gain2/1  "<CurvatureDerivative>"
  Bus Selector1/1 -> Gain7/1  "<Curvature>"
  Bus Selector1/3 -> Gain3/1  "<HeadingAngle>"
  Gain7/1 -> Data Type Conversion/1
  Gain2/1 -> Data Type Conversion1/1
  Gain3/1 -> Data Type Conversion2/1
  Bus Selector1/4 -> Data Type Conversion3/1  "<LateralOffset>"
  Bus Selector1/5 -> Data Type Conversion4/1  "<Strength>"
  Data Type Conversion/1 -> Bus Creator/1  "Curvature"
  Data Type Conversion1/1 -> Bus Creator/2  "CurvatureDerivative"
  Data Type Conversion2/1 -> Bus Creator/3  "HeadingAngle"
  Data Type Conversion3/1 -> Bus Creator/4  "LateralOffset"
  Data Type Conversion4/1 -> Bus Creator/5  "Strength"
  Data Type Conversion9/1 -> Bus Creator1/5  "Strength"
  Data Type Conversion6/1 -> Bus Creator1/2  "CurvatureDerivative"
  Data Type Conversion7/1 -> Bus Creator1/3  "HeadingAngle"
  Data Type Conversion8/1 -> Bus Creator1/4  "LateralOffset"
  Data Type Conversion5/1 -> Bus Creator1/1  "Curvature"
  Bus Selector2/1 -> Gain5/1  "<Curvature>"
  Selector1/1 -> Bus Selector2/1
  Bus Selector2/4 -> Data Type Conversion8/1  "<LateralOffset>"
  Bus Selector2/5 -> Data Type Conversion9/1  "<Strength>"
  Bus Selector2/2 -> Gain1/1  "<CurvatureDerivative>"
  Gain4/1 -> Data Type Conversion7/1
  Gain5/1 -> Data Type Conversion5/1
  Gain1/1 -> Data Type Conversion6/1
  Bus Selector2/3 -> Gain4/1  "<HeadingAngle>"
  Bus Creator2/1 -> Out/1
  Bus Creator/1 -> Bus Creator2/1  "Left"
  Bus Creator1/1 -> Bus Creator2/2  "Right"
  Bus Selector1/6 -> Matrix Concatenate/2  "<CurveLength>"
  Bus Selector1/7 -> Data Type Conversion11/1  "<BoundaryType>"
  Data Type Conversion10/1 -> Bus Creator/6  "XExtent"
  Data Type Conversion11/1 -> Bus Creator/7  "BoundaryType"
  Data Type Conversion12/1 -> Bus Creator1/6  "XExtent"
  Data Type Conversion13/1 -> Bus Creator1/7  "BoundaryType"
  Bus Selector2/7 -> Data Type Conversion13/1  "<BoundaryType>"
  Matrix Concatenate/1 -> Data Type Conversion10/1
  Constant/1 -> Matrix Concatenate/1
  Matrix Concatenate1/1 -> Data Type Conversion12/1
  Bus Selector2/6 -> Matrix Concatenate1/2  "<CurveLength>"
  Constant1/1 -> Matrix Concatenate1/1

== matlab function HighwayLaneFollowingTestBench/Vision Detector Variant/Probabilistic Detection Sensor/Pack Measurements  ==
  data: u input; y output Bus: BusVision; structInit parameter; measurementNoise parameter
function y = fcn(u,structInit,measurementNoise)

y = structInit;
y.NumDetections = u.NumDetections;
y.IsValidTime = u.IsValidTime;
for n = 1:u.NumDetections
    y.Detections(n).Time = u.Detections(n).Time;
    y.Detections(n).Measurement = u.Detections(n).Measurement(1:3);
    y.Detections(n).MeasurementNoise = measurementNoise;
    y.Detections(n).SensorIndex = u.Detections(n).SensorIndex;
    y.Detections(n).ObjectClassID = u.Detections(n).ObjectClassID;
    y.Detections(n).ObjectAttributes = u.Detections(n).ObjectAttributes;
    y.Detections(n).MeasurementParameters = u.Detections(n).MeasurementParameters;
    y.Detections(n).MeasurementParameters.HasVelocity = false;
end

== matlab function HighwayLaneFollowingTestBench/Vehicle Dynamics/Pack Ego Actor ==
  data: pos input; a output Bus: BusVehiclePose size=1; vel input; yaw input; yawRate input
function a = packEgo(pos,vel,yaw,yawRate)
% Pack ego information into a single ego actor bus
%
% Important note:
% Output is a bus of type BusVehiclePose. This bus must match the bus 
% elements expected by Scenario Reader. You can view the 
% bus association using 'Edit Data' in the menu above.

a = struct(...
    'ActorID',1,...
    'Position', [pos(1) pos(2) 0], ...
    'Velocity', [vel(1) vel(2) 0], ...
    'Roll', 0, ...
    'Pitch', 0, ...
    'Yaw', yaw, ...
    'AngularVelocity', [0 0 yawRate]);

== matlab function HighwayLaneFollowingTestBench/Metrics Assessment/Collision Detection/Detect Collision ==
  data: actors input; collision output; vehicleProfiles parameter
function collision = detectCollision(actors, vehicleProfiles)

% Associate on-path MATLAB function
coder.extrinsic('helperSLDetectVehicleCollision');

% Assign default value to define output data type
collision = false;

% Call on-path MATLAB function
collision = helperSLDetectVehicleCollision(actors.Actors, vehicleProfiles);

== matlab function HighwayLaneFollowingTestBench/Metrics Assessment/Collision Detection/Detect MIO ==
  data: actors input; mioIndex output; mioRelLongDist output; mioRelLongVel output; lane input; headway output; vehicleProfiles parameter
function [mioIndex,mioRelLongDist,mioRelLongVel,headway] = detectMIO(actors,lane,vehicleProfiles)

% Find the closest vehicle in ego lane
longDist = zeros(1,actors.NumActors);
for i = 1:actors.NumActors
    
    % Positions with respect to ego
    x = actors.Actors(i).Position(1);
    y = actors.Actors(i).Position(2);
    
    % Default longitudinal distance from vehicle
    longDist(i) = inf;
    
    % Check if vehicle is ahead of ego
    if x >= 0
        % Find left lane coordinates closest to vehicle position x
        [~,n] = min(abs(lane.LaneBoundaries(1).Coordinates(:,1)-x));
        yleftLane = lane.LaneBoundaries(1).Coordinates(n,2);

        % Find right lane coordinates closest to vehicle position x
        [~,n] = min(abs(lane.LaneBoundaries(2).Coordinates(:,1)-x));
        yrightLane = lane.LaneBoundaries(2).Coordinates(n,2);

        % Check if vehicle is in same lane as ego
        if (yrightLane <= y) && (y <= yleftLane)
            longDist(i) = x;
        end       
    end
end

% Minimum distance between vehicle rear axles
[minLongDist,mioIndex] = min(longDist);

if isempty(minLongDist) || isinf(minLongDist)
    mioIndex = nan;
    mioRelLongDist = inf;
    mioRelLongVel = inf;
    headway = inf;
else
    mioRelLongDist = minLongDist;
    mioRelLongVel = actors.Actors(mioIndex).Velocity(1);
    headway = headwayLongDist(minLongDist,mioIndex,vehicleProfiles);
end

end

function headway = headwayLongDist(dist,mioIndex,vehicleProfiles)
% Longitudinal headway is distance between vehicle rear axles
% reduced by distance of ego rear axle to front and 
% reduced by distance of MIO rear axle to rear

% Notes on origin offset
% - Origin offset is the relative position [x,yz] of vehicle center with 
%   respect to the rear axle
% - Distance rear axle center to vehicle center = negative of origin offset(1)

% Ego distance from rear axle to front
egoProfile = vehicleProfiles(1);
egoDistRearAxleToVehCenter = - egoProfile.OriginOffset(1);
egoDistRearAxleToFront = egoProfile.Length/2 + egoDistRearAxleToVehCenter;

% MIO distance from rear axle to rear
mioProfile = vehicleProfiles(mioIndex);
mioDistRearAxleToVehCenter = - mioProfile.OriginOffset(1);
mioDistRearAxleToRear = mioProfile.Length/2 - mioDistRearAxleToVehCenter;

% Longitudinal headway is distance from front of ego to rear of MIO
headway = dist - egoDistRearAxleToFront - mioDistRearAxleToRear;

end

== matlab function HighwayLaneFollowingTestBench/Vision Detector Variant/Probabilistic Detection Sensor/Rear Axle to Vehicle Center ==
  data: u input; y output Bus: LaneSensor; offsetX parameter
function y = fcn(u,offsetX)
% Shift detections to vehicle center as required by lateral controller

y.Left  = shiftLateralOffset(u.Left,  offsetX);
y.Right = shiftLateralOffset(u.Right, offsetX);

end

function lane = shiftLateralOffset(lane, offsetX)
if lane.Strength > 0
    
    % Polynomial coefficients from curvature
    p = [lane.Curvature/2,...
         lane.HeadingAngle,...
         lane.LateralOffset];
     
    % Update lateral offset
    lane.LateralOffset(:) = polyval(p, offsetX);
end
end
